simulink model "Final_EWASP_VC"  (R2022a)
settings: Solver=ode1  StartTime=0.0  StopTime=24*3600  FixedStep=10  RelTol=1e-3
values from neighbouring files (symbols this model uses):
  Aux_Threshold = 52    [Setup_Code_EWASP_VC.m]
  buildingAge = 2005    [Setup_Code_EWASP_VC.m]
  ceilingHeight = 2.4    [Setup_Code_EWASP_VC.m]
  conductiveHconnectMatrix = [ ... (first row only)    [Setup_Code_EWASP_VC.m]
  cRoofGreen = 100000    [Setup_Code_EWASP_VC.m]
  Defrost_After_Time = 30    [Setup_Code_EWASP_VC.m]
  DHWDemandProfile = occFreegainHotwaterElecTestPassiveOcc3(:,3)    [Setup_Code_EWASP_VC.m]
  Elec_Max = Elec_Max*(30/24.2)    [Setup_Code_EWASP_VC.m]
  Elec_Mid = Elec_Mid*(30/24.2)    [Setup_Code_EWASP_VC.m]
  Elec_Min = Elec_Min*(30/24.2)    [Setup_Code_EWASP_VC.m]
  ElecDemandProfile = occFreegainHotwaterElecTestPassiveOcc3(:,4)    [Setup_Code_EWASP_VC.m]
  ElecFixed = [Elec_Max(6,2) Elec_Max(6,4) Elec_Max(6,6) Elec_Max(6,7) ... (first row only)    [Setup_Code_EWASP_VC.m]
  floorOrCeilingArea = floorOrCeilingArea*1.15    [Setup_Code_EWASP_VC.m]
  forceCold = 0    [Setup_Code_EWASP_VC.m]
  freegain = occFreegainHotwaterElecTestPassiveOcc3(:,2)-max(occupancy)*25    [Setup_Code_EWASP_VC.m]
  furnitureModelOn = 1    [Setup_Code_EWASP_VC.m]
  Heat_Max = Heat_Max*(30/24.2)    [Setup_Code_EWASP_VC.m]
  Heat_Mid = Heat_Mid*(30/24.2)    [Setup_Code_EWASP_VC.m]
  Heat_Min = Heat_Min*(30/24.2)    [Setup_Code_EWASP_VC.m]
  HeatFixed = [Heat_Max(6,2) Heat_Max(6,4) Heat_Max(6,6) Heat_Max(6,7) ... (first row only)    [Setup_Code_EWASP_VC.m]
  HeatingOnProfile = repmat(HeatingOnProfile,365,1)    [Setup_Code_EWASP_VC.m]
  HEX_ReturnLowerLimit = 52.5    [Setup_Code_EWASP_VC.m]
  HEX_ReturnUpperLimit = 55    [Setup_Code_EWASP_VC.m]
  LeakMultiplier = 1+(2*(rand()-0.5)/10)    [Setup_Code_EWASP_VC.m]
  loopCap = 15    [Setup_Code_EWASP_VC.m]
  maxOcc = max(occupancyProfile)    [Setup_Code_EWASP_VC.m]
  NESW_wallArea = max(NESW_Lengths*ceilingHeight-NESW_Windows,0)    [Setup_Code_EWASP_VC.m]
  NESW_Windows = [ ... (first row only)    [Setup_Code_EWASP_VC.m]
  numRooms = roomCount    [Setup_Code_EWASP_VC.m]
  offsetDays = 0    [Setup_Code_EWASP_VC.m]
  pumpChoice = pumpChoices(MinIndex,1)    [Setup_Code_EWASP_VC.m]
  pumpRamp = 180    [Setup_Code_EWASP_VC.m]
  ReturnLowerLimit = 37.5    [Setup_Code_EWASP_VC.m]
  ReturnUpperLimit = 40    [Setup_Code_EWASP_VC.m]
  RoofIrradiance = Flat_NS_EW_RoofIrradiance(:,1)    [Setup_Code_EWASP_VC.m]
  roofStartTemp = ones(11,1)*20    [Setup_Code_EWASP_VC.m]
  rooftype = 0    [Setup_Code_EWASP_VC.m]
  RoomDataMatrix = [zeros(1,12);ones(1,12)*wallDensity;zeros(1,12);ones(1,12)*wallU;ones(1,12)*windowU;ones(1,12)*floorU;ones(1,12)*ceilingU;zeros(1,12);windowArea, 0;floorOrCeilingArea;zeros(1,12);floorOrCeilingArea*ceilingHeight]    [Setup_Code_EWASP_VC.m]
  roomVol = roomVol*1.15    [Setup_Code_EWASP_VC.m]
  slabStartTemp = (GroundTempTimeSeries(offsetDays*1440+1,1)+thermostatSetting)/2    [Setup_Code_EWASP_VC.m]
  SlackRequest = zeros(1440,1)    [Setup_Code_EWASP_VC.m]
  SolarThermalExists = 0    [Setup_Code_EWASP_VC.m]
  SourceFixed = HeatFixed-ElecFixed    [Setup_Code_EWASP_VC.m]
  StateSeries = StateSeriesGenerator(22,7,1)    [Setup_Code_EWASP_VC.m]
  Tank_Lower_Temp = 49.5    [Setup_Code_EWASP_VC.m]
  Tank_Upper_Temp = 52    [Setup_Code_EWASP_VC.m]
  Tank_Volume_m3 = 0.15    [Setup_Code_EWASP_VC.m]
  TankHeatHour = randi([1 5])-1    [Setup_Code_EWASP_VC.m]
  thermostatSetting = 20.0    (= 20)    [Setup_Code_EWASP_VC.m]
  upDown = [0;0;0;0;1;1;1;1;1;1;1]    [Setup_Code_EWASP_VC.m]
  variableASHP = 1    [Setup_Code_EWASP_VC.m]
  wallStartTempExt = thermostatSetting*(0.266+0.00215*outdoorStartTemp+0.018*wallU+0.00113*outdoorStartTemp*wallU+0.0068*wallU^2)    [Setup_Code_EWASP_VC.m]
undefined symbols (not defined in the file or in its folder): a, ceilingU, condUDMatrix, convUDMatrix, deltaPEXPANDED_E, deltaPEXPANDED_E2, deltaPEXPANDED_N, deltaPEXPANDED_N2, deltaPEXPANDED_S, deltaPEXPANDED_S2, deltaPEXPANDED_W, deltaPEXPANDED_W2, DesiredDHWTemp, DesiredFlowTempVsInOutDeltaTemp, DiffuseHorizontal, DiscIntNeverNeededParam, DNI, dwnAndConcrete, DWORK_A_HX, DWORK_CHK_FLU, DWORK_CP_NODE, DWORK_DH, DWORK_FLUID, DWORK_HCON, DWORK_LOSS, DWORK_MDOTDOWN, DWORK_MDOTIN, DWORK_MDOTUP, DWORK_MIX, DWORK_PRESS, DWORK_QDOTIN, DWORK_RHO_NODE, DWORK_TIN, DWORK_TS_OLD, DWORK_V_NODE, GroundTempTimeSeries, HCM, HCM2, HCM_closed, HCM_closed2, intermediateU, IsTop, massFlowMatrix, neighbourMatrix, numericalRoomUse, RadiatorMatrix, room2roomflowmatrix_E, room2roomflowmatrix_E2, room2roomflowmatrix_N, room2roomflowmatrix_N2, room2roomflowmatrix_S, room2roomflowmatrix_S2, room2roomflowmatrix_W, room2roomflowmatrix_W2, StateAirInEXPANDED_E, StateAirInEXPANDED_E2, StateAirInEXPANDED_N, StateAirInEXPANDED_N2, StateAirInEXPANDED_S, StateAirInEXPANDED_S2 ... (+23)
libraries: simulink x6, dspsigops x4, dspmtrx3 x4, carnot x3, spsEdgeDetectorLib x2, dspstat3 x2, powerlib_meascontrol x1, simulink_extras x1
(part 26 of 27)

== matlab function Final_EWASP_VC/Subsystem_Room11/Bathroom/furniture/MATLAB Function ==
  data: roomArea input; woodPlasticHeatTransfertoroom output; roomtype input; roomTemp input; TemperatureWoodPlastic input; TemperatureSoft input; deltaTWoodPlasticMean output; softHeatTransfertoroom output; deltaTsoftMean output
function [woodPlasticHeatTransfertoroom,deltaTWoodPlasticMean,softHeatTransfertoroom,deltaTsoftMean]=FurnitureTransfer(roomArea,roomtype,roomTemp,TemperatureWoodPlastic,TemperatureSoft)

excessMeanWoodPlastic=TemperatureWoodPlastic-roomTemp;
excessMeanSoft=TemperatureSoft-roomTemp;

if roomtype==1
    
%carpetMass=roomArea*2.041;% 2.041kg/m2 based on  https://thecarpetstop.co.uk/buying-guides/#:~:text=These%20are%20given%20in%20ounces,commonly%20a%20more%20luxurious%20carpet.  
%underlayMass=roomArea*2.7;% 2.7kg/m2 based on https://www.carpet-underlay-shop.co.uk/products/duralay-durafit-650-15-07m2-from-5-74-per-m2
CurtainMass=15;
Sofafabricmass=10;% based on 2lb/ft^3 and 2 sofas - 3 seater and 2 seater https://furnitureblog.simplicitysofas.com/blog/what-is-the-difference-between-a-sofa-cushions-foam-density-and-firmness/ 
matressMass=0; %no beds
duvetandSheetsMass=0; %no beds

SoftMass=CurtainMass+Sofafabricmass;
woodPlasticMass=roomArea*20-SoftMass;

elseif roomtype ==2

%carpetMass=roomArea*2.041;% 2.041kg/m2 based on  https://thecarpetstop.co.uk/buying-guides/#:~:text=These%20are%20given%20in%20ounces,commonly%20a%20more%20luxurious%20carpet.  
%underlayMass=roomArea*2.7;% 2.7kg/m2 based on https://www.carpet-underlay-shop.co.uk/products/duralay-durafit-650-15-07m2-from-5-74-per-m2
CurtainMass=15;
matressMass=40; %https://democracy.york.gov.uk/documents/s2116/Annex%20C%20REcycling%20Report%20frnweights2005.pdf
duvetandSheetsMass=5; %5kg based on %https://inthewash.co.uk/washing-machines/can-you-wash-a-king-size-duvet-in-an-8-9-10-kg-washing-machine/#:~:text=A%20king%20size%20duvet%20will,able%20to%20cope%20with%20them.
Sofafabricmass=0; %no sofa

SoftMass=CurtainMass+matressMass+duvetandSheetsMass;


woodPlasticMass=roomArea*30-SoftMass;
woodPlasticMass=roomArea*30-SoftMass;

else %room is other e.g. kitchen - assume heavily furnished, and majority wood or plastic
    
CurtainMass=0; %
matressMass=0; %
duvetandSheetsMass=0; %
Sofafabricmass=0; %no sofa

SoftMass=0;

woodPlasticMass=roomArea*35-SoftMass;
woodPlasticMass=roomArea*35-SoftMass;    
    
end





softDensityA=60;
softDensityB=80;
softThicknessA=0.15; %represents thicker furnishings (sofa foam etc.)
softThicknessB=0.01; %Represents thinner funishings (e.g. carpet)

SoftMassA=duvetandSheetsMass+Sofafabricmass+matressMass;
SoftMassB=CurtainMass;

SoftVolumeA=SoftMassA/softDensityA;
SoftVolumeB=SoftMassA/softDensityB;

approxSoftA_SA=(SoftVolumeA/softThicknessA);%no 2* here due to one surface usually being obscured
approxSoftB_SA=(SoftVolumeB/softThicknessB);%as above

Softradius=3*((SoftVolumeA+SoftVolumeB)/(approxSoftA_SA+approxSoftB_SA));
SoftbiotNumber=(10/0.03)*((SoftVolumeA+SoftVolumeB)/(approxSoftA_SA+approxSoftB_SA));% appropriate for typical soft furnishings with conductivity 0.03 w/mK and convective transfer coefficient 10 W/k m2 
SoftFBI=1/(0.282*SoftbiotNumber+0.944);
excessSurfSoft=SoftFBI*excessMeanSoft;
softHeatTransfertoroom=excessSurfSoft*10*(approxSoftA_SA+approxSoftB_SA);
deltaTsoftMean=-softHeatTransfertoroom/(softDensityA*SoftVolumeA*1400+softDensityB*SoftVolumeB*1400);

if isnan(deltaTsoftMean)==1
deltaTsoftMean=0;
else
end
    
woodPlasticDensity=800; %600kg/m^3 as of Influence of internal thermal mass on the indoor thermal dynamics and integration of phase change materials in furniture for building energy storage: A review
woodPlasticThickness=0.018; %0.018m typical as of as of Influence of internal thermal mass on the indoor thermal dynamics and integration of phase change materials in furniture for building energy storage: A review
woodPlasticVolume=woodPlasticMass/woodPlasticDensity;
approxWoodPlasticSA=(woodPlasticVolume/woodPlasticThickness); %a rough surface area calculation for the wooden elements

radius=3*woodPlasticVolume/approxWoodPlasticSA;
biotNumber=(10/0.2)*(woodPlasticVolume/approxWoodPlasticSA);% appropriate for typical wood with conductivity 0.2 w/mK and convective transfer coefficient 10 W/k m2 
FBI=1/(0.282*biotNumber+0.944);
excessSurfWoodPlastic=FBI*excessMeanWoodPlastic;
woodPlasticHeatTransfertoroom=excessSurfWoodPlastic*10*approxWoodPlasticSA;
deltaTWoodPlasticMean=-woodPlasticHeatTransfertoroom/(800*woodPlasticVolume*1700);% heat capacity of wodd and plastic is assumer 1700 J/Kg, they are very close in capacity anyway (1.76 wood, 1.67 plastic)

deltaTWoodPlasticMean(isnan(deltaTWoodPlasticMean))=0;

softHeatTransfertoroom(isnan(softHeatTransfertoroom))=0;

%end

== matlab function Final_EWASP_VC/Subsystem3/MATLAB Function1 ==
  data: u input; y output
function y = fcn(u)

u(isnan(u))=0;
u(isinf(u))=0;
y=u;

== matlab function Final_EWASP_VC/Subsystem3/MATLAB Function2 ==
  data: u input; y output
function y = fcn(u)

u(isnan(u))=0;
u(isinf(u))=0;
y=u;

== matlab function Final_EWASP_VC/Subsystem3/MATLAB Function3 ==
  data: u input; y output
function y = fcn(u)

u(isnan(u))=0;
u(isinf(u))=0;
y=u;

== matlab function Final_EWASP_VC/Subsystem3/MATLAB Function4 ==
  data: u input; y output
function y = fcn(u)

u(isnan(u))=0;
u(isinf(u))=0;
y=u;

== matlab function Final_EWASP_VC/MATLAB Function2 ==
  data: A_COLL input; delta_T_Panel output; Q_SOLAR input; T_panel input; T_amb input; T_inlet input; m_dot input; T_outlet output
function [delta_T_Panel,T_outlet]  = fcn(A_COLL,Q_SOLAR,T_panel,T_amb,T_inlet,m_dot)



c=[3.5*A_COLL
    0.02*A_COLL
    0
    0
    7000
    0];

optical_efficiency=0.8;

    T_diff = (T_panel - T_amb); % difference between mean collector temperature and ambient */
	POWER = 2.0*m_dot*4180*(T_panel - T_inlet); %this is the heat lost from the panel energy due to flow of water in and out of the panel, the 2 arises due to transforming (Tout-Tin) to (2Tm-2Tin) using Tout=2Tm-Tin

    
    delta_T_Panel = ((Q_SOLAR*A_COLL)*optical_efficiency - T_diff *(c(1,1) + c(2,1)*T_diff)-POWER) / (c(5,1)*A_COLL);
    T_outlet=2*T_panel-T_inlet;

== matlab function Final_EWASP_VC/MATLAB Function3 ==
  data: T_bottom_Tank input; solarHeatToWater output; T_diff input; mDotPanel input; Hex_Temp input; Hex_Uval input; coilWaterMass input; dT_HEXsolar output
function [solarHeatToWater,dT_HEXsolar] = fcn(T_bottom_Tank,T_diff,mDotPanel,Hex_Temp,Hex_Uval,coilWaterMass)


CondTrans=((Hex_Temp-T_bottom_Tank)*Hex_Uval)/(coilWaterMass*4180);
minCondTrans=-abs(Hex_Temp-T_bottom_Tank);
maxCondTrans=abs(Hex_Temp-T_bottom_Tank);

CondTrans=min(max(minCondTrans,CondTrans),maxCondTrans);


solarHeatToWater=CondTrans*(coilWaterMass*4180);

ConvTrans=T_diff*mDotPanel/coilWaterMass;
dT_HEXsolar=ConvTrans-CondTrans;

== matlab function Final_EWASP_VC/ASHP_Subsystem_Variable/Subsystem/Calc Qdotfortemp ==
  data: refSendTemp input; RequiredQDot output; actReturnTemp input; massFlowTotal input
function RequiredQDot = fcn(refSendTemp,actReturnTemp,massFlowTotal)

RequiredQDot=massFlowTotal*4180*(refSendTemp-actReturnTemp)/1000;

RequiredQDot(isnan(RequiredQDot))=0;

== matlab function Final_EWASP_VC/ASHP_Subsystem_Variable/Subsystem/MATLAB Function1 ==
  data: mDot input; DeltaTPump output; QDot input
function DeltaTPump = fcn(mDot,QDot)

%mFlowSide=10;

DeltaTPump=(QDot/(mDot*4180));
DeltaTPump(isnan(DeltaTPump))=0;
DeltaTPump(isinf(DeltaTPump))=0;

== matlab function Final_EWASP_VC/Subsystem_Room6/Bedroom1/Subsystem1/MATLAB Function ==
  data: uValWall input; deltaTint output; c_InPU input; c_MidPU input; c_OutPU input; T_InWallNEWS input; T_MidWallNEWS input; T_OutWallNEWS input; T_Room input; T_AmbientSeries input; windSpeedSeries input; deltaTmid output; deltaTout output; NESW_wallArea input; roomNumber input; logRoomHeatLoss output; Time input; offsetDays input
function [deltaTint,deltaTmid,deltaTout,logRoomHeatLoss] = fcn(uValWall,c_InPU,c_MidPU,c_OutPU,T_InWallNEWS, T_MidWallNEWS,T_OutWallNEWS,T_Room,T_AmbientSeries,windSpeedSeries,NESW_wallArea,roomNumber,Time,offsetDays)




  deltaTint=zeros(1,4);
   deltaTmid=zeros(1,4);
    deltaTout=zeros(1,4);
    logRoomHeatLoss=zeros(1,4);

    v_Wind=windSpeedSeries(ceil((offsetDays*1440)+Time/60+0.00001),1);
   T_Ambient=T_AmbientSeries(ceil((offsetDays*1440)+Time/60+0.00001),1);
    
k_InMid=uValWall*2;
k_OutMid=uValWall*2;


NEWS_wallArea=NESW_wallArea;
NEWS_wallArea([3 4],:)=NEWS_wallArea([4 3],:);
RoomWallAreas_NEWS=NEWS_wallArea(:,roomNumber)';


for i=1:4
    
    if RoomWallAreas_NEWS(1,i)>0

c_In=c_InPU*RoomWallAreas_NEWS(1,i);
c_Mid=c_MidPU*RoomWallAreas_NEWS(1,i);
c_Out=c_OutPU*RoomWallAreas_NEWS(1,i);

T_InWall=T_InWallNEWS(1,i);
T_MidWall=T_MidWallNEWS(1,i);
T_OutWall=T_OutWallNEWS(1,i);
    
aA=[-(k_InMid*RoomWallAreas_NEWS(1,i))/c_In (k_InMid*RoomWallAreas_NEWS(1,i))/c_In 0
 (k_InMid*RoomWallAreas_NEWS(1,i))/c_Mid -((k_InMid+k_OutMid)*RoomWallAreas_NEWS(1,i))/c_Mid (k_OutMid*RoomWallAreas_NEWS(1,i))/c_Mid
 0 (k_OutMid*RoomWallAreas_NEWS(1,i))/c_Out -(k_OutMid*RoomWallAreas_NEWS(1,i))/c_Out];

bA=[1/c_In 0 0
 0 1/c_Mid 0
 0 0 1/c_Out];
    
ab=[T_InWall
    T_MidWall
    T_OutWall];

bb=[(2.5*(T_Room-T_InWall)+5.6*(T_Room-T_InWall))*RoomWallAreas_NEWS(1,i)
0    
(2.8+3*v_Wind)*(T_Ambient-T_OutWall)+5.6*(T_Ambient-T_OutWall)*RoomWallAreas_NEWS(1,i)];

deltaT=aA*ab+bA*bb;

    deltaTint(1,i)=deltaT(1,1);
   deltaTmid(1,i)=deltaT(2,1);
    deltaTout(1,i)=deltaT(3,1);
    
    logRoomHeatLoss(1,i)=bb(1,1);
    
    else
        
        deltaTint(1,i)=0;
   deltaTmid(1,i)=0;
    deltaTout(1,i)=0;
        
    logRoomHeatLoss(1,i)=0;
    
    end
    
end

== matlab function Final_EWASP_VC/Subsystem_Room6/Bedroom1/Subsystem1/MATLAB Function1 ==
  data: PU_AreaIrradianceTotal output; angleSeries input; NEWS_Irradiance output; DNISeries input; DiffSeries input; Time input; offsetDays input; SurfaceAlbedo input; NESW_wallArea input; roomNumber input; c_OutPU input; deltaTexternalNEWS output
function [PU_AreaIrradianceTotal, NEWS_Irradiance,deltaTexternalNEWS] = SolarSeriesToExtWallGains(angleSeries,DNISeries,DiffSeries,Time,offsetDays,SurfaceAlbedo,NESW_wallArea,roomNumber,c_OutPU)

%deltaTexternalNEWS=zeros(1,4);

Angle_NEWS=angleSeries(ceil((offsetDays*1440)+Time/60+0.00001),1:4);
DNI=DNISeries(ceil((offsetDays*1440)+Time/60+0.00001),1);

PU_AreaDiff=DiffSeries(ceil((offsetDays*1440)+Time/60+0.00001),1)/2;%extracts correct Diff for the timestep, factor of 1/2 corrects for 90 degree walls (so only half Diff irradiance can be utilised)
PU_AreaDNI=cos(deg2rad(Angle_NEWS))*DNI;
NEWS_wallArea=NESW_wallArea;
NEWS_wallArea([3 4],:)=NEWS_wallArea([4 3],:);

RoomWallAreas_NEWS=NEWS_wallArea(:,roomNumber)';
PU_AreaIrradianceTotal=(PU_AreaDNI+PU_AreaDiff)*(1-SurfaceAlbedo);

NEWS_Irradiance=RoomWallAreas_NEWS.*PU_AreaIrradianceTotal;
deltaTexternalNEWS=NEWS_Irradiance./(c_OutPU*RoomWallAreas_NEWS);

for i=1:4
   
    if RoomWallAreas_NEWS(1,i)==0
        deltaTexternalNEWS(1,i)=0;
    else
        
    end
    
end

== matlab function Final_EWASP_VC/Subsystem_Room8/Bedroom3/Subsystem1/MATLAB Function ==
  data: uValWall input; deltaTint output; c_InPU input; c_MidPU input; c_OutPU input; T_InWallNEWS input; T_MidWallNEWS input; T_OutWallNEWS input; T_Room input; T_AmbientSeries input; windSpeedSeries input; deltaTmid output; deltaTout output; NESW_wallArea input; roomNumber input; logRoomHeatLoss output; Time input; offsetDays input
function [deltaTint,deltaTmid,deltaTout,logRoomHeatLoss] = fcn(uValWall,c_InPU,c_MidPU,c_OutPU,T_InWallNEWS, T_MidWallNEWS,T_OutWallNEWS,T_Room,T_AmbientSeries,windSpeedSeries,NESW_wallArea,roomNumber,Time,offsetDays)




  deltaTint=zeros(1,4);
   deltaTmid=zeros(1,4);
    deltaTout=zeros(1,4);
    logRoomHeatLoss=zeros(1,4);

    v_Wind=windSpeedSeries(ceil((offsetDays*1440)+Time/60+0.00001),1);
   T_Ambient=T_AmbientSeries(ceil((offsetDays*1440)+Time/60+0.00001),1);
    
k_InMid=uValWall*2;
k_OutMid=uValWall*2;


NEWS_wallArea=NESW_wallArea;
NEWS_wallArea([3 4],:)=NEWS_wallArea([4 3],:);
RoomWallAreas_NEWS=NEWS_wallArea(:,roomNumber)';


for i=1:4
    
    if RoomWallAreas_NEWS(1,i)>0

c_In=c_InPU*RoomWallAreas_NEWS(1,i);
c_Mid=c_MidPU*RoomWallAreas_NEWS(1,i);
c_Out=c_OutPU*RoomWallAreas_NEWS(1,i);

T_InWall=T_InWallNEWS(1,i);
T_MidWall=T_MidWallNEWS(1,i);
T_OutWall=T_OutWallNEWS(1,i);
    
aA=[-(k_InMid*RoomWallAreas_NEWS(1,i))/c_In (k_InMid*RoomWallAreas_NEWS(1,i))/c_In 0
 (k_InMid*RoomWallAreas_NEWS(1,i))/c_Mid -((k_InMid+k_OutMid)*RoomWallAreas_NEWS(1,i))/c_Mid (k_OutMid*RoomWallAreas_NEWS(1,i))/c_Mid
 0 (k_OutMid*RoomWallAreas_NEWS(1,i))/c_Out -(k_OutMid*RoomWallAreas_NEWS(1,i))/c_Out];

bA=[1/c_In 0 0
 0 1/c_Mid 0
 0 0 1/c_Out];
    
ab=[T_InWall
    T_MidWall
    T_OutWall];

bb=[(2.5*(T_Room-T_InWall)+5.6*(T_Room-T_InWall))*RoomWallAreas_NEWS(1,i)
0    
(2.8+3*v_Wind)*(T_Ambient-T_OutWall)+5.6*(T_Ambient-T_OutWall)*RoomWallAreas_NEWS(1,i)];

deltaT=aA*ab+bA*bb;

    deltaTint(1,i)=deltaT(1,1);
   deltaTmid(1,i)=deltaT(2,1);
    deltaTout(1,i)=deltaT(3,1);
    
    logRoomHeatLoss(1,i)=bb(1,1);
    
    else
        
        deltaTint(1,i)=0;
   deltaTmid(1,i)=0;
    deltaTout(1,i)=0;
        
    logRoomHeatLoss(1,i)=0;
    
    end
    
end

== matlab function Final_EWASP_VC/Subsystem_Room8/Bedroom3/Subsystem1/MATLAB Function1 ==
  data: PU_AreaIrradianceTotal output; angleSeries input; NEWS_Irradiance output; DNISeries input; DiffSeries input; Time input; offsetDays input; SurfaceAlbedo input; NESW_wallArea input; roomNumber input; c_OutPU input; deltaTexternalNEWS output
function [PU_AreaIrradianceTotal, NEWS_Irradiance,deltaTexternalNEWS] = SolarSeriesToExtWallGains(angleSeries,DNISeries,DiffSeries,Time,offsetDays,SurfaceAlbedo,NESW_wallArea,roomNumber,c_OutPU)

%deltaTexternalNEWS=zeros(1,4);

Angle_NEWS=angleSeries(ceil((offsetDays*1440)+Time/60+0.00001),1:4);
DNI=DNISeries(ceil((offsetDays*1440)+Time/60+0.00001),1);

PU_AreaDiff=DiffSeries(ceil((offsetDays*1440)+Time/60+0.00001),1)/2;%extracts correct Diff for the timestep, factor of 1/2 corrects for 90 degree walls (so only half Diff irradiance can be utilised)
PU_AreaDNI=cos(deg2rad(Angle_NEWS))*DNI;
NEWS_wallArea=NESW_wallArea;
NEWS_wallArea([3 4],:)=NEWS_wallArea([4 3],:);

RoomWallAreas_NEWS=NEWS_wallArea(:,roomNumber)';
PU_AreaIrradianceTotal=(PU_AreaDNI+PU_AreaDiff)*(1-SurfaceAlbedo);

NEWS_Irradiance=RoomWallAreas_NEWS.*PU_AreaIrradianceTotal;
deltaTexternalNEWS=NEWS_Irradiance./(c_OutPU*RoomWallAreas_NEWS);

for i=1:4
   
    if RoomWallAreas_NEWS(1,i)==0
        deltaTexternalNEWS(1,i)=0;
    else
        
    end
    
end

== matlab function Final_EWASP_VC/Subsystem_Room9/Bedroom4/Subsystem1/MATLAB Function ==
  data: uValWall input; deltaTint output; c_InPU input; c_MidPU input; c_OutPU input; T_InWallNEWS input; T_MidWallNEWS input; T_OutWallNEWS input; T_Room input; T_AmbientSeries input; windSpeedSeries input; deltaTmid output; deltaTout output; NESW_wallArea input; roomNumber input; logRoomHeatLoss output; Time input; offsetDays input
function [deltaTint,deltaTmid,deltaTout,logRoomHeatLoss] = fcn(uValWall,c_InPU,c_MidPU,c_OutPU,T_InWallNEWS, T_MidWallNEWS,T_OutWallNEWS,T_Room,T_AmbientSeries,windSpeedSeries,NESW_wallArea,roomNumber,Time,offsetDays)




  deltaTint=zeros(1,4);
   deltaTmid=zeros(1,4);
    deltaTout=zeros(1,4);
    logRoomHeatLoss=zeros(1,4);

    v_Wind=windSpeedSeries(ceil((offsetDays*1440)+Time/60+0.00001),1);
   T_Ambient=T_AmbientSeries(ceil((offsetDays*1440)+Time/60+0.00001),1);
    
k_InMid=uValWall*2;
k_OutMid=uValWall*2;


NEWS_wallArea=NESW_wallArea;
NEWS_wallArea([3 4],:)=NEWS_wallArea([4 3],:);
RoomWallAreas_NEWS=NEWS_wallArea(:,roomNumber)';


for i=1:4
    
    if RoomWallAreas_NEWS(1,i)>0

c_In=c_InPU*RoomWallAreas_NEWS(1,i);
c_Mid=c_MidPU*RoomWallAreas_NEWS(1,i);
c_Out=c_OutPU*RoomWallAreas_NEWS(1,i);

T_InWall=T_InWallNEWS(1,i);
T_MidWall=T_MidWallNEWS(1,i);
T_OutWall=T_OutWallNEWS(1,i);
    
aA=[-(k_InMid*RoomWallAreas_NEWS(1,i))/c_In (k_InMid*RoomWallAreas_NEWS(1,i))/c_In 0
 (k_InMid*RoomWallAreas_NEWS(1,i))/c_Mid -((k_InMid+k_OutMid)*RoomWallAreas_NEWS(1,i))/c_Mid (k_OutMid*RoomWallAreas_NEWS(1,i))/c_Mid
 0 (k_OutMid*RoomWallAreas_NEWS(1,i))/c_Out -(k_OutMid*RoomWallAreas_NEWS(1,i))/c_Out];

bA=[1/c_In 0 0
 0 1/c_Mid 0
 0 0 1/c_Out];
    
ab=[T_InWall
    T_MidWall
    T_OutWall];

bb=[(2.5*(T_Room-T_InWall)+5.6*(T_Room-T_InWall))*RoomWallAreas_NEWS(1,i)
0    
(2.8+3*v_Wind)*(T_Ambient-T_OutWall)+5.6*(T_Ambient-T_OutWall)*RoomWallAreas_NEWS(1,i)];

deltaT=aA*ab+bA*bb;

    deltaTint(1,i)=deltaT(1,1);
   deltaTmid(1,i)=deltaT(2,1);
    deltaTout(1,i)=deltaT(3,1);
    
    logRoomHeatLoss(1,i)=bb(1,1);
    
    else
        
        deltaTint(1,i)=0;
   deltaTmid(1,i)=0;
    deltaTout(1,i)=0;
        
    logRoomHeatLoss(1,i)=0;
    
    end
    
end

== matlab function Final_EWASP_VC/Subsystem_Room9/Bedroom4/Subsystem1/MATLAB Function1 ==
  data: PU_AreaIrradianceTotal output; angleSeries input; NEWS_Irradiance output; DNISeries input; DiffSeries input; Time input; offsetDays input; SurfaceAlbedo input; NESW_wallArea input; roomNumber input; c_OutPU input; deltaTexternalNEWS output
function [PU_AreaIrradianceTotal, NEWS_Irradiance,deltaTexternalNEWS] = SolarSeriesToExtWallGains(angleSeries,DNISeries,DiffSeries,Time,offsetDays,SurfaceAlbedo,NESW_wallArea,roomNumber,c_OutPU)

%deltaTexternalNEWS=zeros(1,4);

Angle_NEWS=angleSeries(ceil((offsetDays*1440)+Time/60+0.00001),1:4);
DNI=DNISeries(ceil((offsetDays*1440)+Time/60+0.00001),1);

PU_AreaDiff=DiffSeries(ceil((offsetDays*1440)+Time/60+0.00001),1)/2;%extracts correct Diff for the timestep, factor of 1/2 corrects for 90 degree walls (so only half Diff irradiance can be utilised)
PU_AreaDNI=cos(deg2rad(Angle_NEWS))*DNI;
NEWS_wallArea=NESW_wallArea;
NEWS_wallArea([3 4],:)=NEWS_wallArea([4 3],:);

RoomWallAreas_NEWS=NEWS_wallArea(:,roomNumber)';
PU_AreaIrradianceTotal=(PU_AreaDNI+PU_AreaDiff)*(1-SurfaceAlbedo);

NEWS_Irradiance=RoomWallAreas_NEWS.*PU_AreaIrradianceTotal;
deltaTexternalNEWS=NEWS_Irradiance./(c_OutPU*RoomWallAreas_NEWS);

for i=1:4
   
    if RoomWallAreas_NEWS(1,i)==0
        deltaTexternalNEWS(1,i)=0;
    else
        
    end
    
end

== matlab function Final_EWASP_VC/Subsystem_Room10/En suite/Subsystem1/MATLAB Function ==
  data: uValWall input; deltaTint output; c_InPU input; c_MidPU input; c_OutPU input; T_InWallNEWS input; T_MidWallNEWS input; T_OutWallNEWS input; T_Room input; T_AmbientSeries input; windSpeedSeries input; deltaTmid output; deltaTout output; NESW_wallArea input; roomNumber input; logRoomHeatLoss output; Time input; offsetDays input
function [deltaTint,deltaTmid,deltaTout,logRoomHeatLoss] = fcn(uValWall,c_InPU,c_MidPU,c_OutPU,T_InWallNEWS, T_MidWallNEWS,T_OutWallNEWS,T_Room,T_AmbientSeries,windSpeedSeries,NESW_wallArea,roomNumber,Time,offsetDays)




  deltaTint=zeros(1,4);
   deltaTmid=zeros(1,4);
    deltaTout=zeros(1,4);
    logRoomHeatLoss=zeros(1,4);

    v_Wind=windSpeedSeries(ceil((offsetDays*1440)+Time/60+0.00001),1);
   T_Ambient=T_AmbientSeries(ceil((offsetDays*1440)+Time/60+0.00001),1);
    
k_InMid=uValWall*2;
k_OutMid=uValWall*2;


NEWS_wallArea=NESW_wallArea;
NEWS_wallArea([3 4],:)=NEWS_wallArea([4 3],:);
RoomWallAreas_NEWS=NEWS_wallArea(:,roomNumber)';


for i=1:4
    
    if RoomWallAreas_NEWS(1,i)>0

c_In=c_InPU*RoomWallAreas_NEWS(1,i);
c_Mid=c_MidPU*RoomWallAreas_NEWS(1,i);
c_Out=c_OutPU*RoomWallAreas_NEWS(1,i);

T_InWall=T_InWallNEWS(1,i);
T_MidWall=T_MidWallNEWS(1,i);
T_OutWall=T_OutWallNEWS(1,i);
    
aA=[-(k_InMid*RoomWallAreas_NEWS(1,i))/c_In (k_InMid*RoomWallAreas_NEWS(1,i))/c_In 0
 (k_InMid*RoomWallAreas_NEWS(1,i))/c_Mid -((k_InMid+k_OutMid)*RoomWallAreas_NEWS(1,i))/c_Mid (k_OutMid*RoomWallAreas_NEWS(1,i))/c_Mid
 0 (k_OutMid*RoomWallAreas_NEWS(1,i))/c_Out -(k_OutMid*RoomWallAreas_NEWS(1,i))/c_Out];

bA=[1/c_In 0 0
 0 1/c_Mid 0
 0 0 1/c_Out];
    
ab=[T_InWall
    T_MidWall
    T_OutWall];

bb=[(2.5*(T_Room-T_InWall)+5.6*(T_Room-T_InWall))*RoomWallAreas_NEWS(1,i)
0    
(2.8+3*v_Wind)*(T_Ambient-T_OutWall)+5.6*(T_Ambient-T_OutWall)*RoomWallAreas_NEWS(1,i)];

deltaT=aA*ab+bA*bb;

    deltaTint(1,i)=deltaT(1,1);
   deltaTmid(1,i)=deltaT(2,1);
    deltaTout(1,i)=deltaT(3,1);
    
    logRoomHeatLoss(1,i)=bb(1,1);
    
    else
        
        deltaTint(1,i)=0;
   deltaTmid(1,i)=0;
    deltaTout(1,i)=0;
        
    logRoomHeatLoss(1,i)=0;
    
    end
    
end

== matlab function Final_EWASP_VC/Subsystem_Room10/En suite/Subsystem1/MATLAB Function1 ==
  data: PU_AreaIrradianceTotal output; angleSeries input; NEWS_Irradiance output; DNISeries input; DiffSeries input; Time input; offsetDays input; SurfaceAlbedo input; NESW_wallArea input; roomNumber input; c_OutPU input; deltaTexternalNEWS output
function [PU_AreaIrradianceTotal, NEWS_Irradiance,deltaTexternalNEWS] = SolarSeriesToExtWallGains(angleSeries,DNISeries,DiffSeries,Time,offsetDays,SurfaceAlbedo,NESW_wallArea,roomNumber,c_OutPU)

%deltaTexternalNEWS=zeros(1,4);

Angle_NEWS=angleSeries(ceil((offsetDays*1440)+Time/60+0.00001),1:4);
DNI=DNISeries(ceil((offsetDays*1440)+Time/60+0.00001),1);

PU_AreaDiff=DiffSeries(ceil((offsetDays*1440)+Time/60+0.00001),1)/2;%extracts correct Diff for the timestep, factor of 1/2 corrects for 90 degree walls (so only half Diff irradiance can be utilised)
PU_AreaDNI=cos(deg2rad(Angle_NEWS))*DNI;
NEWS_wallArea=NESW_wallArea;
NEWS_wallArea([3 4],:)=NEWS_wallArea([4 3],:);

RoomWallAreas_NEWS=NEWS_wallArea(:,roomNumber)';
PU_AreaIrradianceTotal=(PU_AreaDNI+PU_AreaDiff)*(1-SurfaceAlbedo);

NEWS_Irradiance=RoomWallAreas_NEWS.*PU_AreaIrradianceTotal;
deltaTexternalNEWS=NEWS_Irradiance./(c_OutPU*RoomWallAreas_NEWS);

for i=1:4
   
    if RoomWallAreas_NEWS(1,i)==0
        deltaTexternalNEWS(1,i)=0;
    else
        
    end
    
end

== matlab function Final_EWASP_VC/Subsystem_Room11/Bathroom/Subsystem1/MATLAB Function ==
  data: uValWall input; deltaTint output; c_InPU input; c_MidPU input; c_OutPU input; T_InWallNEWS input; T_MidWallNEWS input; T_OutWallNEWS input; T_Room input; T_AmbientSeries input; windSpeedSeries input; deltaTmid output; deltaTout output; NESW_wallArea input; roomNumber input; logRoomHeatLoss output; Time input; offsetDays input
function [deltaTint,deltaTmid,deltaTout,logRoomHeatLoss] = fcn(uValWall,c_InPU,c_MidPU,c_OutPU,T_InWallNEWS, T_MidWallNEWS,T_OutWallNEWS,T_Room,T_AmbientSeries,windSpeedSeries,NESW_wallArea,roomNumber,Time,offsetDays)




  deltaTint=zeros(1,4);
   deltaTmid=zeros(1,4);
    deltaTout=zeros(1,4);
    logRoomHeatLoss=zeros(1,4);

    v_Wind=windSpeedSeries(ceil((offsetDays*1440)+Time/60+0.00001),1);
   T_Ambient=T_AmbientSeries(ceil((offsetDays*1440)+Time/60+0.00001),1);
    
k_InMid=uValWall*2;
k_OutMid=uValWall*2;


NEWS_wallArea=NESW_wallArea;
NEWS_wallArea([3 4],:)=NEWS_wallArea([4 3],:);
RoomWallAreas_NEWS=NEWS_wallArea(:,roomNumber)';


for i=1:4
    
    if RoomWallAreas_NEWS(1,i)>0

c_In=c_InPU*RoomWallAreas_NEWS(1,i);
c_Mid=c_MidPU*RoomWallAreas_NEWS(1,i);
c_Out=c_OutPU*RoomWallAreas_NEWS(1,i);

T_InWall=T_InWallNEWS(1,i);
T_MidWall=T_MidWallNEWS(1,i);
T_OutWall=T_OutWallNEWS(1,i);
    
aA=[-(k_InMid*RoomWallAreas_NEWS(1,i))/c_In (k_InMid*RoomWallAreas_NEWS(1,i))/c_In 0
 (k_InMid*RoomWallAreas_NEWS(1,i))/c_Mid -((k_InMid+k_OutMid)*RoomWallAreas_NEWS(1,i))/c_Mid (k_OutMid*RoomWallAreas_NEWS(1,i))/c_Mid
 0 (k_OutMid*RoomWallAreas_NEWS(1,i))/c_Out -(k_OutMid*RoomWallAreas_NEWS(1,i))/c_Out];

bA=[1/c_In 0 0
 0 1/c_Mid 0
 0 0 1/c_Out];
    
ab=[T_InWall
    T_MidWall
    T_OutWall];

bb=[(2.5*(T_Room-T_InWall)+5.6*(T_Room-T_InWall))*RoomWallAreas_NEWS(1,i)
0    
(2.8+3*v_Wind)*(T_Ambient-T_OutWall)+5.6*(T_Ambient-T_OutWall)*RoomWallAreas_NEWS(1,i)];

deltaT=aA*ab+bA*bb;

    deltaTint(1,i)=deltaT(1,1);
   deltaTmid(1,i)=deltaT(2,1);
    deltaTout(1,i)=deltaT(3,1);
    
    logRoomHeatLoss(1,i)=bb(1,1);
    
    else
        
        deltaTint(1,i)=0;
   deltaTmid(1,i)=0;
    deltaTout(1,i)=0;
        
    logRoomHeatLoss(1,i)=0;
    
    end
    
end

== matlab function Final_EWASP_VC/Subsystem_Room2/Kitchen/Subsystem1/MATLAB Function ==
  data: uValWall input; deltaTint output; c_InPU input; c_MidPU input; c_OutPU input; T_InWallNEWS input; T_MidWallNEWS input; T_OutWallNEWS input; T_Room input; T_AmbientSeries input; windSpeedSeries input; deltaTmid output; deltaTout output; NESW_wallArea input; roomNumber input; logRoomHeatLoss output; Time input; offsetDays input
function [deltaTint,deltaTmid,deltaTout,logRoomHeatLoss] = fcn(uValWall,c_InPU,c_MidPU,c_OutPU,T_InWallNEWS, T_MidWallNEWS,T_OutWallNEWS,T_Room,T_AmbientSeries,windSpeedSeries,NESW_wallArea,roomNumber,Time,offsetDays)




  deltaTint=zeros(1,4);
   deltaTmid=zeros(1,4);
    deltaTout=zeros(1,4);
    logRoomHeatLoss=zeros(1,4);

    v_Wind=windSpeedSeries(ceil((offsetDays*1440)+Time/60+0.00001),1);
   T_Ambient=T_AmbientSeries(ceil((offsetDays*1440)+Time/60+0.00001),1);
    
k_InMid=uValWall*2;
k_OutMid=uValWall*2;


NEWS_wallArea=NESW_wallArea;
NEWS_wallArea([3 4],:)=NEWS_wallArea([4 3],:);
RoomWallAreas_NEWS=NEWS_wallArea(:,roomNumber)';


for i=1:4
    
    if RoomWallAreas_NEWS(1,i)>0

c_In=c_InPU*RoomWallAreas_NEWS(1,i);
c_Mid=c_MidPU*RoomWallAreas_NEWS(1,i);
c_Out=c_OutPU*RoomWallAreas_NEWS(1,i);

T_InWall=T_InWallNEWS(1,i);
T_MidWall=T_MidWallNEWS(1,i);
T_OutWall=T_OutWallNEWS(1,i);
    
aA=[-(k_InMid*RoomWallAreas_NEWS(1,i))/c_In (k_InMid*RoomWallAreas_NEWS(1,i))/c_In 0
 (k_InMid*RoomWallAreas_NEWS(1,i))/c_Mid -((k_InMid+k_OutMid)*RoomWallAreas_NEWS(1,i))/c_Mid (k_OutMid*RoomWallAreas_NEWS(1,i))/c_Mid
 0 (k_OutMid*RoomWallAreas_NEWS(1,i))/c_Out -(k_OutMid*RoomWallAreas_NEWS(1,i))/c_Out];

bA=[1/c_In 0 0
 0 1/c_Mid 0
 0 0 1/c_Out];
    
ab=[T_InWall
    T_MidWall
    T_OutWall];

bb=[(2.5*(T_Room-T_InWall)+5.6*(T_Room-T_InWall))*RoomWallAreas_NEWS(1,i)
0    
(2.8+3*v_Wind)*(T_Ambient-T_OutWall)+5.6*(T_Ambient-T_OutWall)*RoomWallAreas_NEWS(1,i)];

deltaT=aA*ab+bA*bb;

    deltaTint(1,i)=deltaT(1,1);
   deltaTmid(1,i)=deltaT(2,1);
    deltaTout(1,i)=deltaT(3,1);
    
    logRoomHeatLoss(1,i)=bb(1,1);
    
    else
        
        deltaTint(1,i)=0;
   deltaTmid(1,i)=0;
    deltaTout(1,i)=0;
        
    logRoomHeatLoss(1,i)=0;
    
    end
    
end

== matlab function Final_EWASP_VC/Subsystem_Room11/Bathroom/Subsystem1/MATLAB Function1 ==
  data: PU_AreaIrradianceTotal output; angleSeries input; NEWS_Irradiance output; DNISeries input; DiffSeries input; Time input; offsetDays input; SurfaceAlbedo input; NESW_wallArea input; roomNumber input; c_OutPU input; deltaTexternalNEWS output
function [PU_AreaIrradianceTotal, NEWS_Irradiance,deltaTexternalNEWS] = SolarSeriesToExtWallGains(angleSeries,DNISeries,DiffSeries,Time,offsetDays,SurfaceAlbedo,NESW_wallArea,roomNumber,c_OutPU)

%deltaTexternalNEWS=zeros(1,4);

Angle_NEWS=angleSeries(ceil((offsetDays*1440)+Time/60+0.00001),1:4);
DNI=DNISeries(ceil((offsetDays*1440)+Time/60+0.00001),1);

PU_AreaDiff=DiffSeries(ceil((offsetDays*1440)+Time/60+0.00001),1)/2;%extracts correct Diff for the timestep, factor of 1/2 corrects for 90 degree walls (so only half Diff irradiance can be utilised)
PU_AreaDNI=cos(deg2rad(Angle_NEWS))*DNI;
NEWS_wallArea=NESW_wallArea;
NEWS_wallArea([3 4],:)=NEWS_wallArea([4 3],:);

RoomWallAreas_NEWS=NEWS_wallArea(:,roomNumber)';
PU_AreaIrradianceTotal=(PU_AreaDNI+PU_AreaDiff)*(1-SurfaceAlbedo);

NEWS_Irradiance=RoomWallAreas_NEWS.*PU_AreaIrradianceTotal;
deltaTexternalNEWS=NEWS_Irradiance./(c_OutPU*RoomWallAreas_NEWS);

for i=1:4
   
    if RoomWallAreas_NEWS(1,i)==0
        deltaTexternalNEWS(1,i)=0;
    else
        
    end
    
end

== matlab function Final_EWASP_VC/MATLAB Function ==
  data: clock input; HeatSysIn input; SystemActive output; ExternalIn input; ExternalIn2 input; ModelFeedbackIn input; RelaxBand output; ModelFeedbackOut output; ModelFeedbackIn2 input; ModelFeedbackOut2 output; MonitorOut output; MonitorOut2 output
function [SystemActive,RelaxBand,ModelFeedbackOut,ModelFeedbackOut2,MonitorOut,MonitorOut2] = fcn(clock,HeatSysIn,ExternalIn,ExternalIn2,ModelFeedbackIn,ModelFeedbackIn2)

%INPUTS

%Clock - Inputs current simulation time
%
%HeatSys In - an input taken from the state of the building model e.g. the
%current temperature of one of the rooms, or the temperature of building
%component (e.g. wall or radiator). The user can manually change the input
%as shown in the instruction manual
%
%ExternalIn & ExternalIn2 - Time series inputs that are independent of
%model state, usually used to represent user of grid requests to turn
%systems on and off/ change thermostat settinggs
%
%ModelFeedbackIn & ModelFeedbackIn2 - Used to feed back a variable from the
%previous timestep, useful if updating variables such as State of Charge,
%or if latching a system on or off in a deadband (see example 1)

%OUTPUTS
%
%SystemActive -  variable that the user can control by programming logic in
%this function; deactivates heating system if set to zero, returns full control to
%default logic if set to 1. Routed to a scope in tutorial, Routed to space
%heating control in the real model.
%
%RelaxBand - binary variable that the user can control by programming logic in
%this function; changes the thermostat band to 16-16.1oC in the real model
%if set to 1,(minimum acceptable for thermal comfort) leaves thermostat band alone if set to zero.
%Routed to a scope in tutorial to show binary output.
%
%ModelFeedbackOut & ModelFeedbackOut2 - used to send variable values to the
%next timestep - useful when updating a variable such as state of charge,
%or latching a value when programming an additional thermostat (see example 1)

%% example 1  
%%Program for an additional space thermostat - 1440x1 matrix is used as
%%dummy input to represent temperature variation of the building component
%%(e.g. room/radiator) that we are controlling on

if HeatSysIn > 35  %e.g. if temp of chosen building compenent exceeds 20oC

SystemActive = 0; %switch off heating/keep heating off
ModelFeedbackOut=SystemActive; %send value to feedback out, so if temp is within deadband at next step, we can latch to the previous systemActive value

elseif HeatSysIn < 34 %if temp of chosen building compenent falls below 18oC

SystemActive = 1; %switch on heating/keep heating on
ModelFeedbackOut=SystemActive; %send value to feedback out, so if temp is within deadband at next step, we can latch to the previous systemActive value
    
else %if temp is within deadband
    
SystemActive = ModelFeedbackIn; %Latch to previous value i.e. if heating was on, keep it on, and vice versa
ModelFeedbackOut=SystemActive; %send value to feedback out, so if temp is within deadband at next step, we can latch to the previous systemActive value
    
end



%% example 2
%%use an externalIn array to read a value from a 1440x1 (1 element for each minute) binary vector
%%that reduces the thermostat temperature at times of high demand -
%%potentially useful for reduction in peak electricity demand

 
if ExternalIn == 1 %e.g. if external value is 1, which suggests band should be relaxed

RelaxBand=1; %Relax the space heating hysteresis band so that ower temps are acceptable

else

RelaxBand=0; %allow Heating System to continue running

end
% 
% %% example 3
% %%charge a battery at 500W whenever a charge signal is recieved from the
% %%1440x1 vector assigned to input 'ExternalIn1'
% 
% if clock == 0 %simulation is just starting
%     
%     StateOfCharge_J=0; %initialize SoC to zero
%     ModelFeedbackOut2=StateOfCharge_J; %output for net timestep
%     MonitorOut=StateOfCharge_J;
% else
% 
% if ExternalIn2 == 1 && ModelFeedbackIn2 <7200000 %charge signal is being sent and store has not met 2kW limit
%     
%     StateOfCharge_J=ModelFeedbackIn2+500*5; %Charge Store at 500W (*5 accounts for 5 second timestep used by the model)
%     ModelFeedbackOut2=StateOfCharge_J; %output new SoC
%     MonitorOut=StateOfCharge_J;
% else
%     ModelFeedbackOut2=ModelFeedbackIn2; %State of Charge output is same as last timestep
%     MonitorOut=ModelFeedbackOut2;
% end
% end
% 
% MonitorOut2=0; %set unused output to a fixed value

MonitorOut=0;
MonitorOut2=0;
ModelFeedbackOut2=0;

== matlab function Final_EWASP_VC/Subsystem_Room11/Bathroom/Subsystem2/MATLAB Function ==
  data: windowTempsNEWS_in input; deltaT_win_in output; windowTempsNEWS_out input; NESW_Windows input; roomTemp input; outdoorTemp input; absorbedNEWS input; windowUval input; roomNumber input; deltaT_win_out output; Q_to_room output
function [deltaT_win_in,deltaT_win_out,Q_to_room] = fcn(windowTempsNEWS_in,windowTempsNEWS_out,NESW_Windows,roomTemp,outdoorTemp,absorbedNEWS,windowUval,roomNumber)


winAreaNEWS=NESW_Windows;
winAreaNEWS([3 4],:)=winAreaNEWS([4 3],:);
winAreaNEWS=winAreaNEWS(:,roomNumber);

%pane thickness=4mm, density=2500 kg/m^3, heat capacity=840 J/kg

Q_win_in=transpose(absorbedNEWS)/2+windowUval*winAreaNEWS.*(windowTempsNEWS_out-windowTempsNEWS_in)-2.5*winAreaNEWS.*(windowTempsNEWS_in-roomTemp);
Q_win_out=transpose(absorbedNEWS)/2+windowUval*winAreaNEWS.*(windowTempsNEWS_in-windowTempsNEWS_out)-2.5*winAreaNEWS.*(windowTempsNEWS_out-outdoorTemp);
deltaT_win_in=Q_win_in./((0.004*winAreaNEWS)*2500*840);
deltaT_win_out=Q_win_out./((0.004*winAreaNEWS)*2500*840);
Q_to_room=2.5*winAreaNEWS.*(windowTempsNEWS_in-roomTemp);
Q_to_room(isnan(Q_to_room))=0;

== matlab function Final_EWASP_VC/Subsystem_Room9/Bedroom4/Subsystem4/MATLAB Function ==
  data: windowTempsNEWS_in input; deltaT_win_in output; windowTempsNEWS_out input; NESW_Windows input; roomTemp input; outdoorTemp input; absorbedNEWS input; windowUval input; roomNumber input; deltaT_win_out output; Q_to_room output
function [deltaT_win_in,deltaT_win_out,Q_to_room] = fcn(windowTempsNEWS_in,windowTempsNEWS_out,NESW_Windows,roomTemp,outdoorTemp,absorbedNEWS,windowUval,roomNumber)


winAreaNEWS=NESW_Windows;
winAreaNEWS([3 4],:)=winAreaNEWS([4 3],:);
winAreaNEWS=winAreaNEWS(:,roomNumber);

%pane thickness=4mm, density=2500 kg/m^3, heat capacity=840 J/kg

Q_win_in=transpose(absorbedNEWS)/2+windowUval*winAreaNEWS.*(windowTempsNEWS_out-windowTempsNEWS_in)-2.5*winAreaNEWS.*(windowTempsNEWS_in-roomTemp);
Q_win_out=transpose(absorbedNEWS)/2+windowUval*winAreaNEWS.*(windowTempsNEWS_in-windowTempsNEWS_out)-2.5*winAreaNEWS.*(windowTempsNEWS_out-outdoorTemp);
deltaT_win_in=Q_win_in./((0.004*winAreaNEWS)*2500*840);
deltaT_win_out=Q_win_out./((0.004*winAreaNEWS)*2500*840);
Q_to_room=2.5*winAreaNEWS.*(windowTempsNEWS_in-roomTemp);
Q_to_room(isnan(Q_to_room))=0;

== matlab function Final_EWASP_VC/Subsystem_Room5/Landing/Subsystem2/MATLAB Function ==
  data: uValWall input; deltaTint output; c_InPU input; c_MidPU input; c_OutPU input; T_InWallNEWS input; T_MidWallNEWS input; T_OutWallNEWS input; T_Room input; T_AmbientSeries input; windSpeedSeries input; deltaTmid output; deltaTout output; NESW_wallArea input; roomNumber input; logRoomHeatLoss output; Time input; offsetDays input
function [deltaTint,deltaTmid,deltaTout,logRoomHeatLoss] = fcn(uValWall,c_InPU,c_MidPU,c_OutPU,T_InWallNEWS, T_MidWallNEWS,T_OutWallNEWS,T_Room,T_AmbientSeries,windSpeedSeries,NESW_wallArea,roomNumber,Time,offsetDays)




  deltaTint=zeros(1,4);
   deltaTmid=zeros(1,4);
    deltaTout=zeros(1,4);
    logRoomHeatLoss=zeros(1,4);

    v_Wind=windSpeedSeries(ceil((offsetDays*1440)+Time/60+0.00001),1);
   T_Ambient=T_AmbientSeries(ceil((offsetDays*1440)+Time/60+0.00001),1);
    
k_InMid=uValWall*2;
k_OutMid=uValWall*2;


NEWS_wallArea=NESW_wallArea;
NEWS_wallArea([3 4],:)=NEWS_wallArea([4 3],:);
RoomWallAreas_NEWS=NEWS_wallArea(:,roomNumber)';


for i=1:4
    
    if RoomWallAreas_NEWS(1,i)>0

c_In=c_InPU*RoomWallAreas_NEWS(1,i);
c_Mid=c_MidPU*RoomWallAreas_NEWS(1,i);
c_Out=c_OutPU*RoomWallAreas_NEWS(1,i);

T_InWall=T_InWallNEWS(1,i);
T_MidWall=T_MidWallNEWS(1,i);
T_OutWall=T_OutWallNEWS(1,i);
    
aA=[-(k_InMid*RoomWallAreas_NEWS(1,i))/c_In (k_InMid*RoomWallAreas_NEWS(1,i))/c_In 0
 (k_InMid*RoomWallAreas_NEWS(1,i))/c_Mid -((k_InMid+k_OutMid)*RoomWallAreas_NEWS(1,i))/c_Mid (k_OutMid*RoomWallAreas_NEWS(1,i))/c_Mid
 0 (k_OutMid*RoomWallAreas_NEWS(1,i))/c_Out -(k_OutMid*RoomWallAreas_NEWS(1,i))/c_Out];

bA=[1/c_In 0 0
 0 1/c_Mid 0
 0 0 1/c_Out];
    
ab=[T_InWall
    T_MidWall
    T_OutWall];

bb=[(2.5*(T_Room-T_InWall)+5.6*(T_Room-T_InWall))*RoomWallAreas_NEWS(1,i)
0    
(2.8+3*v_Wind)*(T_Ambient-T_OutWall)+5.6*(T_Ambient-T_OutWall)*RoomWallAreas_NEWS(1,i)];

deltaT=aA*ab+bA*bb;

    deltaTint(1,i)=deltaT(1,1);
   deltaTmid(1,i)=deltaT(2,1);
    deltaTout(1,i)=deltaT(3,1);
    
    logRoomHeatLoss(1,i)=bb(1,1);
    
    else
        
        deltaTint(1,i)=0;
   deltaTmid(1,i)=0;
    deltaTout(1,i)=0;
        
    logRoomHeatLoss(1,i)=0;
    
    end
    
end

== matlab function Final_EWASP_VC/Subsystem_Room1/Lounge//Dining/Subsystem2/MATLAB Function2 ==
  data: Angle_NEWS output; angleSeries input; NEWS_DNI output; DNISeries input; DiffSeries input; Time input; offsetDays input; NESW_Windows input; roomNumber input; NEWS_Diff output
function [Angle_NEWS,NEWS_DNI,NEWS_Diff] = SolarSeriesDataExtractor(angleSeries,DNISeries,DiffSeries,Time,offsetDays,NESW_Windows,roomNumber)

%deltaTexternalNEWS=zeros(1,4);

Angle_NEWS=angleSeries(ceil((offsetDays*1440)+Time/60+0.00001),1:4);
DNI=DNISeries(ceil((offsetDays*1440)+Time/60+0.00001),1);
Diff=DiffSeries(ceil((offsetDays*1440)+Time/60+0.00001),1);%extracts correct Diff per unit horizontal area for the timestep (corrected for wall tilt at a later stage

NEWS_windowArea=NESW_Windows;
NEWS_windowArea([3 4],:)=NEWS_windowArea([4 3],:);

RoomWindowAreas_NEWS=NEWS_windowArea(:,roomNumber)';


NEWS_DNI=RoomWindowAreas_NEWS*DNI;
NEWS_Diff=RoomWindowAreas_NEWS*Diff;

== matlab function Final_EWASP_VC/Subsystem_Room3/Utility/Subsystem4/MATLAB Function ==
  data: windowTempsNEWS_in input; deltaT_win_in output; windowTempsNEWS_out input; NESW_Windows input; roomTemp input; outdoorTemp input; absorbedNEWS input; windowUval input; roomNumber input; deltaT_win_out output; Q_to_room output
function [deltaT_win_in,deltaT_win_out,Q_to_room] = fcn(windowTempsNEWS_in,windowTempsNEWS_out,NESW_Windows,roomTemp,outdoorTemp,absorbedNEWS,windowUval,roomNumber)


winAreaNEWS=NESW_Windows;
winAreaNEWS([3 4],:)=winAreaNEWS([4 3],:);
winAreaNEWS=winAreaNEWS(:,roomNumber);

%pane thickness=4mm, density=2500 kg/m^3, heat capacity=840 J/kg

Q_win_in=transpose(absorbedNEWS)/2+windowUval*winAreaNEWS.*(windowTempsNEWS_out-windowTempsNEWS_in)-2.5*winAreaNEWS.*(windowTempsNEWS_in-roomTemp);
Q_win_out=transpose(absorbedNEWS)/2+windowUval*winAreaNEWS.*(windowTempsNEWS_in-windowTempsNEWS_out)-2.5*winAreaNEWS.*(windowTempsNEWS_out-outdoorTemp);
deltaT_win_in=Q_win_in./((0.004*winAreaNEWS)*2500*840);
deltaT_win_out=Q_win_out./((0.004*winAreaNEWS)*2500*840);
Q_to_room=2.5*winAreaNEWS.*(windowTempsNEWS_in-roomTemp);
Q_to_room(isnan(Q_to_room))=0;

== matlab function Final_EWASP_VC/Subsystem_Room4/Hall/Subsystem4/MATLAB Function ==
  data: windowTempsNEWS_in input; deltaT_win_in output; windowTempsNEWS_out input; NESW_Windows input; roomTemp input; outdoorTemp input; absorbedNEWS input; windowUval input; roomNumber input; deltaT_win_out output; Q_to_room output
function [deltaT_win_in,deltaT_win_out,Q_to_room] = fcn(windowTempsNEWS_in,windowTempsNEWS_out,NESW_Windows,roomTemp,outdoorTemp,absorbedNEWS,windowUval,roomNumber)


winAreaNEWS=NESW_Windows;
winAreaNEWS([3 4],:)=winAreaNEWS([4 3],:);
winAreaNEWS=winAreaNEWS(:,roomNumber);

%pane thickness=4mm, density=2500 kg/m^3, heat capacity=840 J/kg

Q_win_in=transpose(absorbedNEWS)/2+windowUval*winAreaNEWS.*(windowTempsNEWS_out-windowTempsNEWS_in)-2.5*winAreaNEWS.*(windowTempsNEWS_in-roomTemp);
Q_win_out=transpose(absorbedNEWS)/2+windowUval*winAreaNEWS.*(windowTempsNEWS_in-windowTempsNEWS_out)-2.5*winAreaNEWS.*(windowTempsNEWS_out-outdoorTemp);
deltaT_win_in=Q_win_in./((0.004*winAreaNEWS)*2500*840);
deltaT_win_out=Q_win_out./((0.004*winAreaNEWS)*2500*840);
Q_to_room=2.5*winAreaNEWS.*(windowTempsNEWS_in-roomTemp);
Q_to_room(isnan(Q_to_room))=0;

== matlab function Final_EWASP_VC/Subsystem_Room6/Bedroom1/Subsystem2/MATLAB Function ==
  data: windowTempsNEWS_in input; deltaT_win_in output; windowTempsNEWS_out input; NESW_Windows input; roomTemp input; outdoorTemp input; absorbedNEWS input; windowUval input; roomNumber input; deltaT_win_out output; Q_to_room output
function [deltaT_win_in,deltaT_win_out,Q_to_room] = fcn(windowTempsNEWS_in,windowTempsNEWS_out,NESW_Windows,roomTemp,outdoorTemp,absorbedNEWS,windowUval,roomNumber)


winAreaNEWS=NESW_Windows;
winAreaNEWS([3 4],:)=winAreaNEWS([4 3],:);
winAreaNEWS=winAreaNEWS(:,roomNumber);

%pane thickness=4mm, density=2500 kg/m^3, heat capacity=840 J/kg

Q_win_in=transpose(absorbedNEWS)/2+windowUval*winAreaNEWS.*(windowTempsNEWS_out-windowTempsNEWS_in)-2.5*winAreaNEWS.*(windowTempsNEWS_in-roomTemp);
Q_win_out=transpose(absorbedNEWS)/2+windowUval*winAreaNEWS.*(windowTempsNEWS_in-windowTempsNEWS_out)-2.5*winAreaNEWS.*(windowTempsNEWS_out-outdoorTemp);
deltaT_win_in=Q_win_in./((0.004*winAreaNEWS)*2500*840);
deltaT_win_out=Q_win_out./((0.004*winAreaNEWS)*2500*840);
Q_to_room=2.5*winAreaNEWS.*(windowTempsNEWS_in-roomTemp);
Q_to_room(isnan(Q_to_room))=0;

== matlab function Final_EWASP_VC/Subsystem_Room5/Landing/Subsystem1/MATLAB Function ==
  data: windowTempsNEWS_in input; deltaT_win_in output; windowTempsNEWS_out input; NESW_Windows input; roomTemp input; outdoorTemp input; absorbedNEWS input; windowUval input; roomNumber input; deltaT_win_out output; Q_to_room output
function [deltaT_win_in,deltaT_win_out,Q_to_room] = fcn(windowTempsNEWS_in,windowTempsNEWS_out,NESW_Windows,roomTemp,outdoorTemp,absorbedNEWS,windowUval,roomNumber)


winAreaNEWS=NESW_Windows;
winAreaNEWS([3 4],:)=winAreaNEWS([4 3],:);
winAreaNEWS=winAreaNEWS(:,roomNumber);

%pane thickness=4mm, density=2500 kg/m^3, heat capacity=840 J/kg

Q_win_in=transpose(absorbedNEWS)/2+windowUval*winAreaNEWS.*(windowTempsNEWS_out-windowTempsNEWS_in)-2.5*winAreaNEWS.*(windowTempsNEWS_in-roomTemp);
Q_win_out=transpose(absorbedNEWS)/2+windowUval*winAreaNEWS.*(windowTempsNEWS_in-windowTempsNEWS_out)-2.5*winAreaNEWS.*(windowTempsNEWS_out-outdoorTemp);
deltaT_win_in=Q_win_in./((0.004*winAreaNEWS)*2500*840);
deltaT_win_out=Q_win_out./((0.004*winAreaNEWS)*2500*840);
Q_to_room=2.5*winAreaNEWS.*(windowTempsNEWS_in-roomTemp);
Q_to_room(isnan(Q_to_room))=0;

== matlab function Final_EWASP_VC/Subsystem_Room6/Bedroom1/Subsystem2/MATLAB Function2 ==
  data: Angle_NEWS output; angleSeries input; NEWS_DNI output; DNISeries input; DiffSeries input; Time input; offsetDays input; NESW_Windows input; roomNumber input; NEWS_Diff output
function [Angle_NEWS,NEWS_DNI,NEWS_Diff] = SolarSeriesDataExtractor(angleSeries,DNISeries,DiffSeries,Time,offsetDays,NESW_Windows,roomNumber)

%deltaTexternalNEWS=zeros(1,4);

Angle_NEWS=angleSeries(ceil((offsetDays*1440)+Time/60+0.00001),1:4);
DNI=DNISeries(ceil((offsetDays*1440)+Time/60+0.00001),1);
Diff=DiffSeries(ceil((offsetDays*1440)+Time/60+0.00001),1);%extracts correct Diff per unit horizontal area for the timestep (corrected for wall tilt at a later stage

NEWS_windowArea=NESW_Windows;
NEWS_windowArea([3 4],:)=NEWS_windowArea([4 3],:);

RoomWindowAreas_NEWS=NEWS_windowArea(:,roomNumber)';


NEWS_DNI=RoomWindowAreas_NEWS*DNI;
NEWS_Diff=RoomWindowAreas_NEWS*Diff;

== matlab function Final_EWASP_VC/Subsystem_Room8/Bedroom3/Subsystem4/MATLAB Function ==
  data: windowTempsNEWS_in input; deltaT_win_in output; windowTempsNEWS_out input; NESW_Windows input; roomTemp input; outdoorTemp input; absorbedNEWS input; windowUval input; roomNumber input; deltaT_win_out output; Q_to_room output
function [deltaT_win_in,deltaT_win_out,Q_to_room] = fcn(windowTempsNEWS_in,windowTempsNEWS_out,NESW_Windows,roomTemp,outdoorTemp,absorbedNEWS,windowUval,roomNumber)


winAreaNEWS=NESW_Windows;
winAreaNEWS([3 4],:)=winAreaNEWS([4 3],:);
winAreaNEWS=winAreaNEWS(:,roomNumber);

%pane thickness=4mm, density=2500 kg/m^3, heat capacity=840 J/kg

Q_win_in=transpose(absorbedNEWS)/2+windowUval*winAreaNEWS.*(windowTempsNEWS_out-windowTempsNEWS_in)-2.5*winAreaNEWS.*(windowTempsNEWS_in-roomTemp);
Q_win_out=transpose(absorbedNEWS)/2+windowUval*winAreaNEWS.*(windowTempsNEWS_in-windowTempsNEWS_out)-2.5*winAreaNEWS.*(windowTempsNEWS_out-outdoorTemp);
deltaT_win_in=Q_win_in./((0.004*winAreaNEWS)*2500*840);
deltaT_win_out=Q_win_out./((0.004*winAreaNEWS)*2500*840);
Q_to_room=2.5*winAreaNEWS.*(windowTempsNEWS_in-roomTemp);
Q_to_room(isnan(Q_to_room))=0;
